simulink model "Boat_sim"  (Simulink 7.8)
settings: Solver=FixedStepDiscrete  StartTime=0.0  StopTime=1000  FixedStep=.01  RelTol=1e-3
InitFcn:
  | clear all
  | missions
  | common
  | physical_constants
  | simulation_constants
  | initial_values
  | l2plus
values from neighbouring files (symbols this model uses):
  InitialPoint = 0    [l2plus.m]
  IPStar = 0    [l2plus.m]
  MaxDwnPthStar = 1    [l2plus.m]
  OC2max = 49999    [simulation_constants.m]
  phi_0 = 0    [simulation_constants.m]
  switchDistance = 4    [l2plus.m]
  T_step = 0.01    [common.m]
  tanIntercept = tan( 45*pi/180 )    [l2plus.m]
  TStar = single(4.5)    [l2plus.m]
  Turn2Track = 0    [l2plus.m]
  wheelbase = 3.27    [physical_constants.m]
undefined symbols (not defined in the file or in its folder): DiscIntNeverNeededParam, Earth, figure8_waypoints, sampling_waypoints, test_waypoints, WGS84
libraries: simulink x21, uSimLib x21, instrumentlib x2, aerolibtransform2 x1, aerolibanimutils x1, simulink_need_slupdate x1
(part 1 of 2)
settings Model: Creator=Administrator  LastModifiedBy=Bryant  ExtModeAutoUpdateStatusClock=off  BufferReuse=off
settings DataIOCC: MaxDataPoints=1  SaveOutput=off  SignalLogging=off
settings OptimizationCC: BlockReduction=off  InlineParams=on  UseIntDivNetSlope=on  InlineInvariantSignals=on  BufferReuse=off  InitFltsAndDblsToZero=on  EfficientFloat2IntCast=on  SimCompilerOptimization=On
settings DebuggingCC: ReadBeforeWriteMsg=DisableAll  SaveWithParameterizedLinksMsg=none  UnderspecifiedInitializationDetection=Simplified  UniqueDataStoreMsg=error  AssertControl=DisableAll
settings HardwareCC: ProdBitPerInt=16  ProdBitPerPointer=16  ProdIntDivRoundTo=Zero  ProdEndianess=LittleEndian  ProdWordSize=16  ProdHWDeviceType=Microchip->dsPIC
settings SFSimCC: SimParseCustomCode=off
settings GRTTargetCC: TargetFcnLib=ansi_tfl_tmw.mat

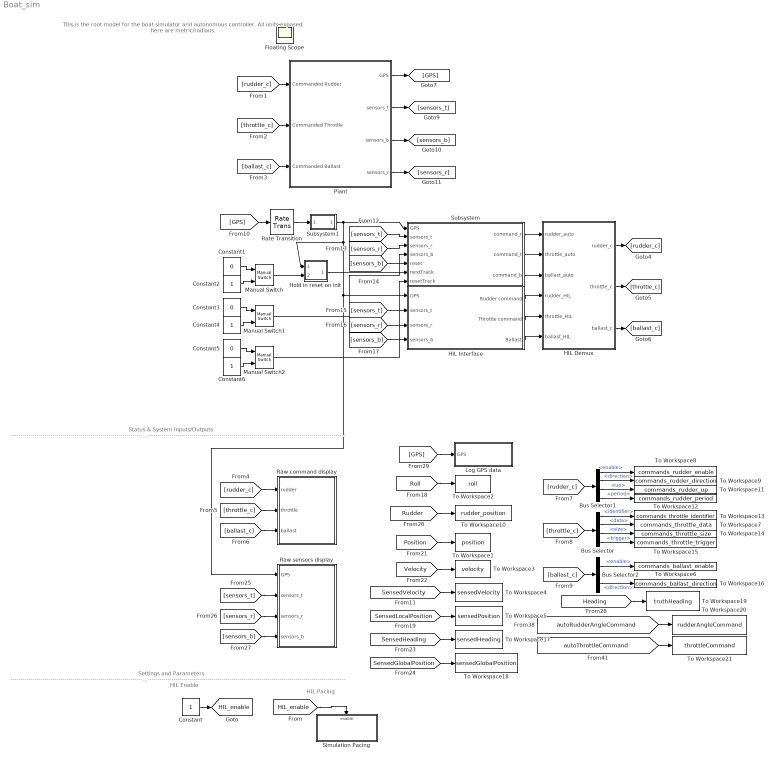
== system Boat_sim ==
  note: This is the root model for the boat simulator and autonomous controller. All
      | units exposed here are metric/radians.
  note: HIL Enable
  note: Settings and Parameters
      | ---------------------------------------------------------------------------------------------------------------------------------------------------------------------------------------------------------------------------------------------------------
  note: HIL Pacing
  note: Status & System Inputs/Outputs
      | ---------------------------------------------------------------------------------------------------------------------------------------------------------------------------------------------------------------------------------------------------------
  Bus Selector : BusSelector  OutputSignals=identifier,data,size,trigger
  Bus Selector1 : BusSelector  OutputSignals=enable,direction,up,period
  Bus Selector2 : BusSelector  OutputSignals=enable,direction
  Constant : Constant  OutDataTypeStr=boolean
  Constant1 : Constant  Value=0  OutDataTypeStr=boolean  SampleTime=Inf
  Constant2 : Constant  OutDataTypeStr=boolean  SampleTime=Inf
  Constant3 : Constant  Value=0  OutDataTypeStr=boolean  SampleTime=Inf
  Constant4 : Constant  OutDataTypeStr=boolean  SampleTime=Inf
  Constant5 : Constant  Value=0  OutDataTypeStr=boolean  SampleTime=Inf
  Constant6 : Constant  OutDataTypeStr=boolean  SampleTime=Inf
  HIL Demux : Subsystem
  HIL Interface : Subsystem
  Hold in reset on init : Subsystem
  Log GPS data : Subsystem
  Manual Switch : simulink/Signal Routing/Manual Switch  sw=1  action=0  varsize=off
  Manual Switch1 : simulink/Signal Routing/Manual Switch  sw=1  action=0  varsize=off
  Manual Switch2 : simulink/Signal Routing/Manual Switch  sw=1  action=0  varsize=off
  Plant : Subsystem
  Rate Transition : RateTransition  OutPortSampleTime=T_step
  Raw command display : Subsystem
  Raw sensors display : Subsystem
  Simulation Pacing : Subsystem  TreatAsAtomicUnit=on
  Subsystem : Subsystem
  Subsystem1 : Subsystem
  To Workspace1 : ToWorkspace  VariableName=position  SampleTime=-1  SaveFormat=Array
  To Workspace10 : ToWorkspace  VariableName=rudder_position  SampleTime=-1  SaveFormat=Array
  To Workspace11 : ToWorkspace  VariableName=commands_rudder_up  SampleTime=-1  SaveFormat=Array
  To Workspace12 : ToWorkspace  VariableName=commands_rudder_period  SampleTime=-1  SaveFormat=Array
  To Workspace13 : ToWorkspace  VariableName=commands_throttle_identifier  SampleTime=-1  SaveFormat=Array
  To Workspace14 : ToWorkspace  VariableName=commands_throttle_size  SampleTime=-1  SaveFormat=Array
  To Workspace15 : ToWorkspace  VariableName=commands_throttle_trigger  SampleTime=-1  SaveFormat=Array
  To Workspace16 : ToWorkspace  VariableName=commands_ballast_direction  SampleTime=-1  SaveFormat=Array
  To Workspace17 : ToWorkspace  VariableName=sensedHeading  SampleTime=-1  SaveFormat=Array
  To Workspace18 : ToWorkspace  VariableName=sensedGlobalPosition  SampleTime=-1  SaveFormat=Array
  To Workspace19 : ToWorkspace  VariableName=truthHeading  SampleTime=-1  SaveFormat=Array
  To Workspace2 : ToWorkspace  VariableName=roll  SampleTime=-1  SaveFormat=Array
  To Workspace20 : ToWorkspace  VariableName=rudderAngleCommand  SampleTime=-1  SaveFormat=Array
  To Workspace21 : ToWorkspace  VariableName=throttleCommand  SampleTime=-1  SaveFormat=Array
  To Workspace3 : ToWorkspace  VariableName=velocity  SampleTime=-1  SaveFormat=Array
  To Workspace4 : ToWorkspace  VariableName=sensedVelocity  SampleTime=-1  SaveFormat=Array
  To Workspace5 : ToWorkspace  VariableName=sensedPosition  SampleTime=-1  SaveFormat=Array
  To Workspace6 : ToWorkspace  VariableName=commands_ballast_enable  SampleTime=-1  SaveFormat=Array
  To Workspace7 : ToWorkspace  VariableName=commands_throttle_data  SampleTime=-1  SaveFormat=Array
  To Workspace8 : ToWorkspace  VariableName=commands_rudder_enable  SampleTime=-1  SaveFormat=Array
  To Workspace9 : ToWorkspace  VariableName=commands_rudder_direction  SampleTime=-1  SaveFormat=Array
  Floating Scope : Scope
      settings: Floating=on
  tag scope: HIL_enable=global
  wires:
  Plant/4(sensors_r) -> [sensors_r]
  Constant/1 -> [HIL_enable]
  Subsystem/1(command_r) -> HIL Demux/1(rudder_auto)
  Subsystem/2(command_t) -> HIL Demux/2(throttle_auto)
  Subsystem/3(command_b) -> HIL Demux/3(ballast_auto)
  [rudder_c] -> Plant/1(Commanded Rudder)
  [throttle_c] -> Plant/2(Commanded Throttle)
  [ballast_c] -> Plant/3(Commanded Ballast)
  Plant/1(GPS) -> [GPS]
  Plant/3(sensors_b) -> [sensors_b]
  Plant/2(sensors_t) -> [sensors_t]
  [sensors_b] -> Subsystem/4(sensors_b)
  [sensors_r] -> Subsystem/3(sensors_r)
  [sensors_t] -> Subsystem/2(sensors_t)
  Constant1/1 -> Manual Switch/1
  Constant2/1 -> Manual Switch/2
  [rudder_c] -> Raw command display/1(rudder)
  [throttle_c] -> Raw command display/2(throttle)
  [ballast_c] -> Raw command display/3(ballast)
  [sensors_t] -> Raw sensors display/2(sensors_t)
  [sensors_r] -> Raw sensors display/3(sensors_r)
  [sensors_b] -> Raw sensors display/4(sensors_b)
  HIL Interface/1(Rudder command) -> HIL Demux/4(rudder_HIL)
  HIL Interface/2(Throttle command) -> HIL Demux/5(throttle_HIL)
  HIL Interface/3(Ballast) -> HIL Demux/6(ballast_HIL)
  HIL Demux/1(rudder_c) -> [rudder_c]
  HIL Demux/3(ballast_c) -> [ballast_c]
  HIL Demux/2(throttle_c) -> [throttle_c]
  [sensors_b] -> HIL Interface/4(sensors_b)
  [sensors_r] -> HIL Interface/3(sensors_r)
  [sensors_t] -> HIL Interface/2(sensors_t)
  [HIL_enable] -> Simulation Pacing/Enable
  [ballast_c] -> Bus Selector2/1
  [Roll] -> To Workspace2/1
  [Rudder] -> To Workspace10/1
  [Position] -> To Workspace1/1
  [throttle_c] -> Bus Selector/1
  Bus Selector/2 -> To Workspace7/1  "<data>"
  [rudder_c] -> Bus Selector1/1
  Bus Selector1/1 -> To Workspace8/1  "<enable>"
  [Velocity] -> To Workspace3/1
  Hold in reset on init/1(Out1) -> Subsystem/5(reset)
  Manual Switch/1 -> Hold in reset on init/2(reset)
  [GPS] -> Rate Transition/1
  Subsystem1/1(GPS+newData) -> Subsystem/1(GPS), Hold in reset on init/1(GPS), HIL Interface/1(GPS), Raw sensors display/1(GPS)
  Constant3/1 -> Manual Switch1/1
  Constant4/1 -> Manual Switch1/2
  Constant5/1 -> Manual Switch2/1
  Constant6/1 -> Manual Switch2/2
  Manual Switch2/1 -> Subsystem/7(resetTrack)
  Manual Switch1/1 -> Subsystem/6(nextTrack)
  [SensedVelocity] -> To Workspace4/1
  [SensedLocalPosition] -> To Workspace5/1
  Bus Selector1/2 -> To Workspace9/1  "<direction>"
  Bus Selector1/3 -> To Workspace11/1  "<up>"
  Bus Selector1/4 -> To Workspace12/1  "<period>"
  Bus Selector/1 -> To Workspace13/1  "<identifier>"
  Bus Selector/3 -> To Workspace14/1  "<size>"
  Bus Selector/4 -> To Workspace15/1  "<trigger>"
  Bus Selector2/1 -> To Workspace6/1  "<enable>"
  Bus Selector2/2 -> To Workspace16/1  "<direction>"
  [SensedHeading] -> To Workspace17/1
  [SensedGlobalPosition] -> To Workspace18/1
  [Heading] -> To Workspace19/1
  [autoRudderAngleCommand] -> To Workspace20/1
  [autoThrottleCommand] -> To Workspace21/1
  [GPS] -> Log GPS data/1(GPS)
  Rate Transition/1 -> Subsystem1/1(GPS)

== system Boat_sim/HIL Demux ==
  rudder_auto : Inport
  throttle_auto : Inport  Port=2
  ballast_auto : Inport  Port=3
  rudder_HIL : Inport  Port=4
  throttle_HIL : Inport  Port=5
  ballast_HIL : Inport  Port=6
  Switch : Switch  Criteria=u2 ~= 0
  Switch1 : Switch  Criteria=u2 ~= 0
  Switch2 : Switch  Criteria=u2 ~= 0
  rudder_c : Outport
  throttle_c : Outport  Port=2
  ballast_c : Outport  Port=3
  wires:
  rudder_HIL/1 -> Switch/1
  [HIL_enable] -> Switch/2, Switch1/2, Switch2/2
  throttle_HIL/1 -> Switch1/1
  ballast_HIL/1 -> Switch2/1
  throttle_auto/1 -> Switch1/3
  rudder_auto/1 -> Switch/3
  ballast_auto/1 -> Switch2/3
  Switch/1 -> rudder_c/1
  Switch1/1 -> throttle_c/1
  Switch2/1 -> ballast_c/1

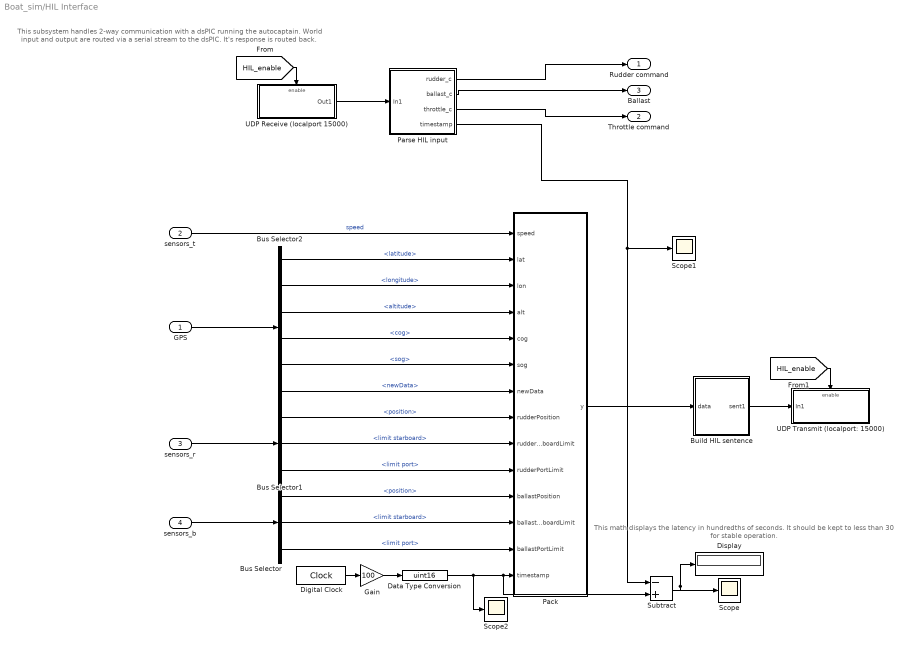
== system Boat_sim/HIL Interface ==
  note: This subsystem handles 2-way communication with a dsPIC running
      | the autocaptain. World input and output are routed via a serial stream
      | to the dsPIC. It's response is routed back.
  note: This math displays the latency in hundredths of seconds.
      | It should be kept to less than 30 for stable operation.
  GPS : Inport
  sensors_t : Inport  Port=2
  sensors_r : Inport  Port=3
  sensors_b : Inport  Port=4
  Build HIL sentence : Subsystem
  Bus Selector : BusSelector  OutputSignals=position,limit starboard,limit port
  Bus Selector1 : BusSelector  OutputSignals=position,limit starboard,limit port
  Bus Selector2 : BusSelector  OutputSignals=latitude,longitude,altitude,cog,sog,newData
  Data Type Conversion : DataTypeConversion  OutDataTypeStr=uint16
  Digital Clock : DigitalClock  SampleTime=.01
  Display : Display
  Gain : Gain  Gain=100
  Pack : MATLAB Function  TreatAsAtomicUnit=on
  Parse HIL input : Subsystem
  Scope : Scope
      settings: YMin=40  YMax=92.5  SaveName=latency  DataFormat=Array
  Scope1 : Scope
      settings: YMin=1470.6  YMax=1625.4  SaveName=latency_in  DataFormat=Array
  Scope2 : Scope
      settings: TimeRange=14  YMin=0  YMax=1400  SaveName=latency_out  DataFormat=Array
  Subtract : Sum  Inputs=-+  OutDataTypeStr=int16
  UDP Receive (localport 15000) : Subsystem  TreatAsAtomicUnit=on
  UDP Transmit (localport: 15000) : Subsystem  TreatAsAtomicUnit=on
  Rudder command : Outport
  Throttle command : Outport  Port=2
  Ballast : Outport  Port=3
  wires:
  UDP Receive (localport 15000)/1(Out1) -> Parse HIL input/1(In1)
  Parse HIL input/2(ballast_c) -> Ballast/1
  Parse HIL input/1(rudder_c) -> Rudder command/1
  sensors_b/1 -> Bus Selector/1
  sensors_r/1 -> Bus Selector1/1
  GPS/1 -> Bus Selector2/1
  Parse HIL input/3(throttle_c) -> Throttle command/1
  Pack/1(y) -> Build HIL sentence/1(data)
  sensors_t/1 -> Pack/1(speed)  "speed"
  Bus Selector2/1 -> Pack/2(lat)  "<latitude>"
  Bus Selector2/2 -> Pack/3(lon)  "<longitude>"
  Bus Selector2/3 -> Pack/4(alt)  "<altitude>"
  Bus Selector2/4 -> Pack/5(cog)  "<cog>"
  Bus Selector2/5 -> Pack/6(sog)  "<sog>"
  [HIL_enable] -> UDP Receive (localport 15000)/Enable
  [HIL_enable] -> UDP Transmit (localport: 15000)/Enable
  Build HIL sentence/1(sent1) -> UDP Transmit (localport: 15000)/1(In1)
  Parse HIL input/4(timestamp) -> Subtract/1, Scope1/1
  Gain/1 -> Data Type Conversion/1
  Digital Clock/1 -> Gain/1
  Data Type Conversion/1 -> Subtract/2, Pack/14(timestamp), Scope2/1
  Subtract/1 -> Scope/1, Display/1
  Bus Selector2/6 -> Pack/7(newData)  "<newData>"
  Bus Selector1/1 -> Pack/8(rudderPosition)  "<position>"
  Bus Selector1/2 -> Pack/9(rudderStarboardLimit)  "<limit starboard>"
  Bus Selector1/3 -> Pack/10(rudderPortLimit)  "<limit port>"
  Bus Selector/1 -> Pack/11(ballastPosition)  "<position>"
  Bus Selector/2 -> Pack/12(ballastStarboardLimit)  "<limit starboard>"
  Bus Selector/3 -> Pack/13(ballastPortLimit)  "<limit port>"

== system Boat_sim/Hold in reset on init ==
  GPS : Inport
  reset : Inport  Port=2
  Bus Selector : BusSelector  OutputSignals=newData
  Compare To Zero : simulink/Logic and Bit Operations/Compare To Zero  relop===  OutDataTypeStr=boolean
  Discrete-Time Integrator : DiscreteIntegrator  SampleTime=-1  LimitOutput=on  UpperSaturationLimit=1  LowerSaturationLimit=0  ICPrevOutput=DiscIntNeverNeededParam  ICPrevScaledInput=DiscIntNeverNeededParam
  Logical Operator : Logic  Operator=OR  AllPortsSameDT=off  OutDataTypeStr=boolean
  Out1 : Outport
  wires:
  Bus Selector/1 -> Discrete-Time Integrator/1  "<newData>"
  Discrete-Time Integrator/1 -> Compare To Zero/1
  Compare To Zero/1 -> Logical Operator/1
  GPS/1 -> Bus Selector/1
  Logical Operator/1 -> Out1/1
  reset/1 -> Logical Operator/2

== system Boat_sim/Log GPS data ==
  GPS : Inport
  Bus Selector3 : BusSelector  OutputSignals=latitude,longitude,altitude,cog,sog
  Mux : Mux  Inputs=3
  To Workspace28 : ToWorkspace  VariableName=globalPosition  SampleTime=-1  SaveFormat=Array
  To Workspace29 : ToWorkspace  VariableName=courseOverGround  SampleTime=-1  SaveFormat=Array
  To Workspace30 : ToWorkspace  VariableName=speedOverGround  SampleTime=-1  SaveFormat=Array
  wires:
  Mux/1 -> To Workspace28/1
  Bus Selector3/1 -> Mux/1  "<latitude>"
  Bus Selector3/2 -> Mux/2  "<longitude>"
  Bus Selector3/3 -> Mux/3  "<altitude>"
  Bus Selector3/4 -> To Workspace29/1  "<cog>"
  Bus Selector3/5 -> To Workspace30/1  "<sog>"
  GPS/1 -> Bus Selector3/1

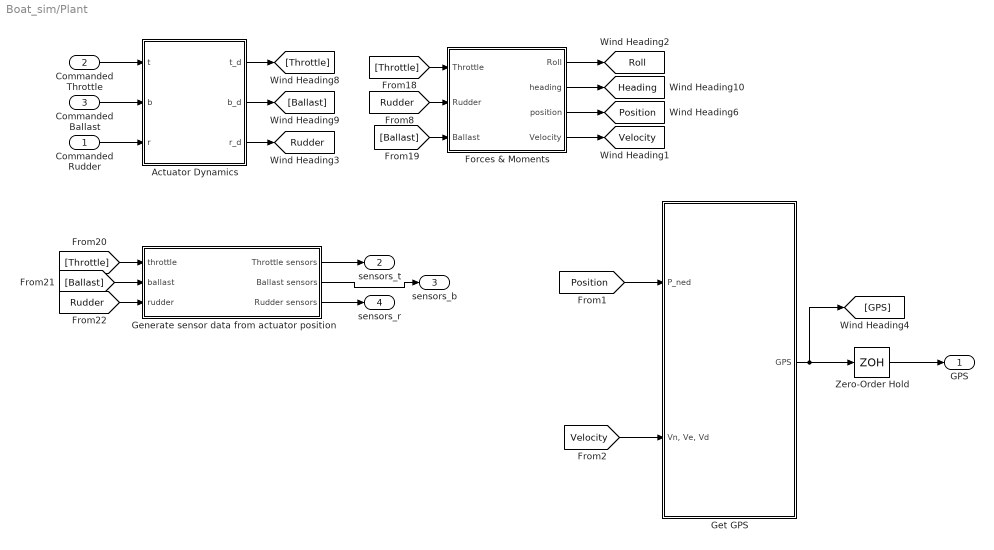
== system Boat_sim/Plant ==
  Commanded Rudder : Inport
  Commanded Throttle : Inport  Port=2
  Commanded Ballast : Inport  Port=3
  Actuator Dynamics : Subsystem
  Forces & Moments : Subsystem
  Generate sensor data from actuator position : Subsystem
  Get GPS : Subsystem
  Zero-Order Hold : ZeroOrderHold  SampleTime=.2
  GPS : Outport
  sensors_t : Outport  Port=2
  sensors_b : Outport  Port=3
  sensors_r : Outport  Port=4
  tag scope: Heading=global, Position=global, Roll=global, Rudder=global, Velocity=global
  wires:
  Commanded Throttle/1 -> Actuator Dynamics/1(t)
  Commanded Rudder/1 -> Actuator Dynamics/3(r)
  Forces & Moments/1(Roll) -> [Roll]
  Commanded Ballast/1 -> Actuator Dynamics/2(b)
  Actuator Dynamics/3(r_d) -> [Rudder]
  [Rudder] -> Forces & Moments/2(Rudder)
  Actuator Dynamics/1(t_d) -> [Throttle]
  [Throttle] -> Forces & Moments/1(Throttle)
  [Ballast] -> Forces & Moments/3(Ballast)
  Actuator Dynamics/2(b_d) -> [Ballast]
  Forces & Moments/2(heading) -> [Heading]
  [Position] -> Get GPS/1(P_ned)
  [Velocity] -> Get GPS/2("Vn, Ve, Vd")
  Get GPS/1(GPS) -> [GPS], Zero-Order Hold/1
  [Rudder] -> Generate sensor data from actuator position/3(rudder)
  [Ballast] -> Generate sensor data from actuator position/2(ballast)
  [Throttle] -> Generate sensor data from actuator position/1(throttle)
  Generate sensor data from actuator position/1(Throttle sensors) -> sensors_t/1
  Generate sensor data from actuator position/2(Ballast sensors) -> sensors_b/1
  Generate sensor data from actuator position/3(Rudder sensors) -> sensors_r/1
  Forces & Moments/4(Velocity) -> [Velocity]
  Forces & Moments/3(position) -> [Position]
  Zero-Order Hold/1 -> GPS/1

== system Boat_sim/Raw command display ==
  rudder : Inport
  throttle : Inport  Port=2
  ballast : Inport  Port=3
  Bus Selector3 : BusSelector  OutputSignals=enable,direction,up,period
  Bus Selector4 : BusSelector  OutputSignals=identifier,data,size,trigger
  Bus Selector5 : BusSelector  OutputSignals=enable,direction
  Display{,1..9} (10 alike) : Display
      Display4 settings: Format=hex (Stored Integer)
      Display5 settings: Format=hex (Stored Integer)
  wires:
  Bus Selector3/4 -> Display3/1  "<period>"
  Bus Selector3/1 -> Display/1  "<enable>"
  Bus Selector3/2 -> Display1/1  "<direction>"
  Bus Selector3/3 -> Display2/1  "<up>"
  Bus Selector4/4 -> Display7/1  "<trigger>"
  Bus Selector4/1 -> Display4/1  "<identifier>"
  Bus Selector4/2 -> Display5/1  "<data>"
  Bus Selector4/3 -> Display6/1  "<size>"
  Bus Selector5/2 -> Display8/1  "<direction>"
  Bus Selector5/1 -> Display9/1  "<enable>"
  rudder/1 -> Bus Selector3/1
  throttle/1 -> Bus Selector4/1
  ballast/1 -> Bus Selector5/1

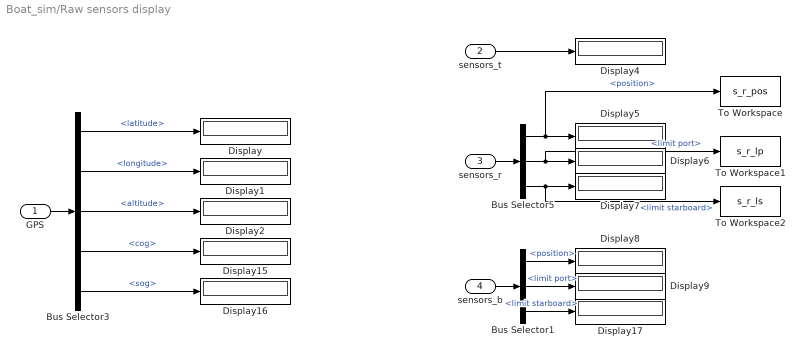
== system Boat_sim/Raw sensors display ==
  GPS : Inport
  sensors_t : Inport  Port=2
  sensors_r : Inport  Port=3
  sensors_b : Inport  Port=4
  Bus Selector1 : BusSelector  OutputSignals=position,limit port,limit starboard
  Bus Selector3 : BusSelector  OutputSignals=latitude,longitude,altitude,cog,sog
  Bus Selector5 : BusSelector  OutputSignals=position,limit port,limit starboard
  Display{,1..2,4..9,15..17} (12 alike) : Display
  To Workspace : ToWorkspace  VariableName=s_r_pos  SampleTime=-1  SaveFormat=Array
  To Workspace1 : ToWorkspace  VariableName=s_r_lp  SampleTime=-1  SaveFormat=Array
  To Workspace2 : ToWorkspace  VariableName=s_r_ls  SampleTime=-1  SaveFormat=Array
  wires:
  Bus Selector3/1 -> Display/1  "<latitude>"
  Bus Selector3/2 -> Display1/1  "<longitude>"
  Bus Selector3/3 -> Display2/1  "<altitude>"
  GPS/1 -> Bus Selector3/1
  sensors_t/1 -> Display4/1
  sensors_r/1 -> Bus Selector5/1
  Bus Selector3/4 -> Display15/1  "<cog>"
  Bus Selector3/5 -> Display16/1  "<sog>"
  sensors_b/1 -> Bus Selector1/1
  Bus Selector5/1 -> Display5/1, To Workspace/1  "<position>"
  Bus Selector5/2 -> Display6/1, To Workspace1/1  "<limit port>"
  Bus Selector5/3 -> Display7/1, To Workspace2/1  "<limit starboard>"
  Bus Selector1/1 -> Display8/1  "<position>"
  Bus Selector1/2 -> Display9/1  "<limit port>"
  Bus Selector1/3 -> Display17/1  "<limit starboard>"

== system Boat_sim/Simulation Pacing ==
  note: This block attempts to lock the simulation down to real-time. This does, however, require that the sim run faster than real time originally,
      | then the Set Pace block sleeps the MATLAB  process to fill up the time til it paces realtime. The number in the display block shouldn't be
      | far from 0 and will probably bounce around both above and below. If it stays substantially below zero (<-.01), then there's a problem as
      | the sim isn't keeping time.
  Enable : EnablePort
  Display1 : Display
      settings: Decimation=20
  Scope : Scope
      settings: SaveName=paceError  DataFormat=Array
  Simulation Pace : aerolibanimutils/Simulation Pace  SimulationPace=1  SleepMode=MATLAB Thread  OutputPaceError=on  SampleTime=T_step
      settings: AttributesFormatString=%<SimulationPace> sec/sec
  wires:
  Simulation Pace/1 -> Display1/1, Scope/1

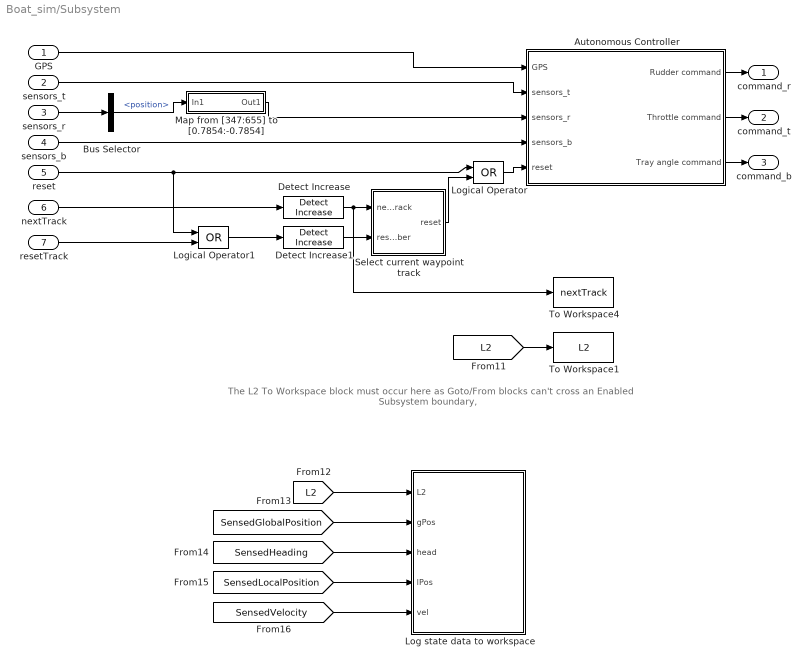
== system Boat_sim/Subsystem ==
  note: The L2 To Workspace block must occur here
      | as Goto/From blocks can't cross an Enabled
      | Subsystem boundary,
  GPS : Inport
  sensors_t : Inport  Port=2
  sensors_r : Inport  Port=3
  sensors_b : Inport  Port=4
  reset : Inport  Port=5
  nextTrack : Inport  Port=6
  resetTrack : Inport  Port=7
  Autonomous Controller : Subsystem  Priority=1
  Bus Selector : BusSelector  OutputSignals=position
  Detect Increase : simulink/Logic and Bit Operations/Detect Increase  vinit=0.0  InputProcessing=Inherited  OutDataTypeStr=boolean
  Detect Increase1 : simulink/Logic and Bit Operations/Detect Increase  vinit=0.0  InputProcessing=Inherited  OutDataTypeStr=boolean
  Log state data to workspace : Subsystem
  Logical Operator : Logic  Operator=OR  AllPortsSameDT=off  OutDataTypeStr=boolean
  Logical Operator1 : Logic  Operator=OR  AllPortsSameDT=off  OutDataTypeStr=boolean
  Map from [347:655] to [0.7854:-0.7854] : Subsystem
  Select current waypoint track : MATLAB Function  TreatAsAtomicUnit=on
  To Workspace1 : ToWorkspace  VariableName=L2  SampleTime=-1  SaveFormat=Array
  To Workspace4 : ToWorkspace  VariableName=nextTrack  SampleTime=-1  SaveFormat=Array
  command_r : Outport
  command_t : Outport  Port=2
  command_b : Outport  Port=3
  wires:
  GPS/1 -> Autonomous Controller/1(GPS)
  Autonomous Controller/1(Rudder command) -> command_r/1
  sensors_t/1 -> Autonomous Controller/2(sensors_t)
  sensors_r/1 -> Bus Selector/1
  Autonomous Controller/2(Throttle command) -> command_t/1
  sensors_b/1 -> Autonomous Controller/4(sensors_b)
  Autonomous Controller/3(Tray angle command) -> command_b/1
  nextTrack/1 -> Detect Increase/1
  Logical Operator/1 -> Autonomous Controller/5(reset)
  Select current waypoint track/1(reset) -> Logical Operator/2
  reset/1 -> Logical Operator/1, Logical Operator1/1
  Detect Increase/1 -> Select current waypoint track/1(nextTrack), To Workspace4/1
  Detect Increase1/1 -> Select current waypoint track/2(resetTrackNumber)
  [L2] -> To Workspace1/1
  Logical Operator1/1 -> Detect Increase1/1
  resetTrack/1 -> Logical Operator1/2
  [SensedVelocity] -> Log state data to workspace/5(vel)
  [L2] -> Log state data to workspace/1(L2)
  [SensedGlobalPosition] -> Log state data to workspace/2(gPos)
  [SensedHeading] -> Log state data to workspace/3(head)
  [SensedLocalPosition] -> Log state data to workspace/4(lPos)
  Map from [347:655] to [0.7854:-0.7854]/1(Out1) -> Autonomous Controller/3(sensors_r)
  Bus Selector/1 -> Map from [347:655] to [0.7854:-0.7854]/1(In1)  "<position>"

== system Boat_sim/Subsystem1 ==
  GPS : Inport
  Bus Assignment : BusAssignment  AssignedSignals=newData
  Data Type Conversion : DataTypeConversion  OutDataTypeStr=boolean
  Pulse Generator : DiscretePulseGenerator  Period=20  PhaseDelay=100  SampleTime=T_step
  GPS+newData : Outport
  wires:
  Pulse Generator/1 -> Data Type Conversion/1
  Data Type Conversion/1 -> Bus Assignment/2
  GPS/1 -> Bus Assignment/1
  Bus Assignment/1 -> GPS+newData/1

== system Boat_sim/HIL Interface/Build HIL sentence ==
  data : Inport
  Bitwise Operator1 : simulink/Logic and Bit Operations/Bitwise Operator  logicop=XOR  UseBitMask=off  BitMask=bin2dec('11011001')  BitMaskRealWorld=Stored Integer
  Constant5 : Constant  Value=37  OutDataTypeStr=uint8
  Constant6 : Constant  Value=38  OutDataTypeStr=uint8
  Constant7 : Constant  Value=94  OutDataTypeStr=uint8
  Constant8 : Constant  Value=38  OutDataTypeStr=uint8
  Constant9 : Constant  OutDataTypeStr=uint8
  Mux3 : Mux  Inputs=3
  Pack : MATLAB Function  TreatAsAtomicUnit=on
  Probe : Probe  ProbeSampleTime=off  ProbeComplexSignal=off  ProbeWidthDataType=uint8
  sent1 : Outport
  wires:
  data/1 -> Probe/1, Mux3/3
  Constant5/1 -> Pack/1(a)
  Constant6/1 -> Pack/2(b)
  Pack/1(y) -> sent1/1
  Mux3/1 -> Bitwise Operator1/1, Pack/3(c)
  Probe/1 -> Mux3/2
  Constant7/1 -> Pack/4(d)
  Constant8/1 -> Pack/5(e)
  Bitwise Operator1/1 -> Pack/6(f)
  Constant9/1 -> Mux3/1

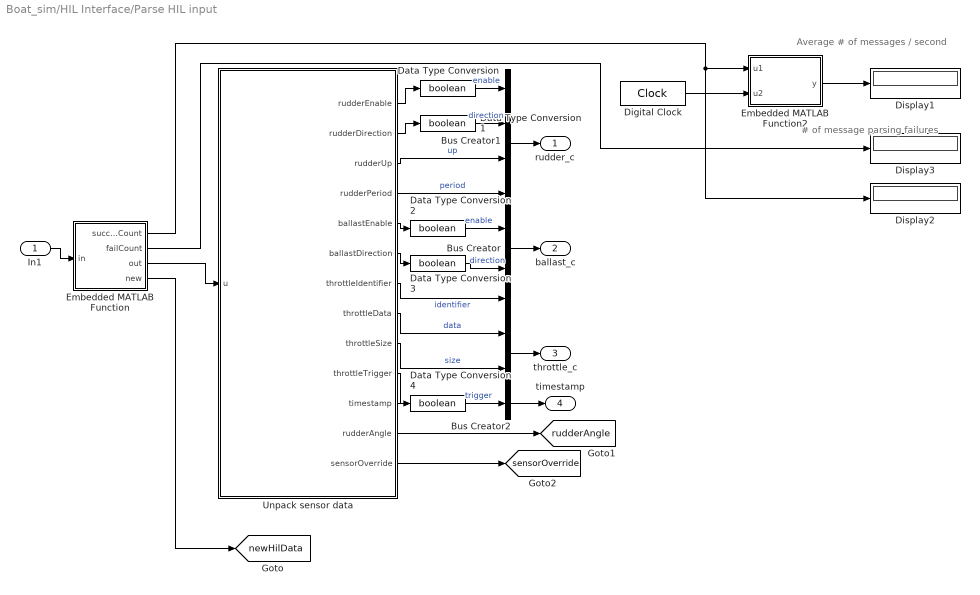
== system Boat_sim/HIL Interface/Parse HIL input ==
  note: # of message parsing failures
  note: Average # of messages / second
  In1 : Inport
  Bus Creator : BusCreator  Inputs=2
  Bus Creator1 : BusCreator
  Bus Creator2 : BusCreator
  Data Type Conversion{,1..4} (5 alike) : DataTypeConversion  OutDataTypeStr=boolean
  Digital Clock : DigitalClock  SampleTime=T_step
  Display1 : Display
  Display2 : Display
  Display3 : Display
  Embedded MATLAB Function : MATLAB Function  TreatAsAtomicUnit=on
  Embedded MATLAB Function2 : MATLAB Function  TreatAsAtomicUnit=on
  Unpack sensor data : MATLAB Function  TreatAsAtomicUnit=on
  rudder_c : Outport
  ballast_c : Outport  Port=2
  throttle_c : Outport  Port=3
  timestamp : Outport  Port=4
  tag scope: newHilData=global, rudderAngle=global, sensorOverride=global
  wires:
  Embedded MATLAB Function/3(out) -> Unpack sensor data/1(u)
  Bus Creator1/1 -> rudder_c/1
  In1/1 -> Embedded MATLAB Function/1(in)
  Bus Creator/1 -> ballast_c/1
  Bus Creator2/1 -> throttle_c/1
  Unpack sensor data/1(rudderEnable) -> Data Type Conversion/1
  Unpack sensor data/2(rudderDirection) -> Data Type Conversion1/1
  Unpack sensor data/3(rudderUp) -> Bus Creator1/3  "up"
  Unpack sensor data/4(rudderPeriod) -> Bus Creator1/4  "period"
  Unpack sensor data/5(ballastEnable) -> Data Type Conversion2/1
  Unpack sensor data/6(ballastDirection) -> Data Type Conversion3/1
  Unpack sensor data/7(throttleIdentifier) -> Bus Creator2/1  "identifier"
  Unpack sensor data/8(throttleData) -> Bus Creator2/2  "data"
  Unpack sensor data/9(throttleSize) -> Bus Creator2/3  "size"
  Unpack sensor data/10(throttleTrigger) -> Data Type Conversion4/1
  Unpack sensor data/11(timestamp) -> timestamp/1
  Embedded MATLAB Function/1(successCount) -> Embedded MATLAB Function2/1(u1), Display2/1
  Digital Clock/1 -> Embedded MATLAB Function2/2(u2)
  Embedded MATLAB Function2/1(y) -> Display1/1
  Data Type Conversion/1 -> Bus Creator1/1  "enable"
  Data Type Conversion1/1 -> Bus Creator1/2  "direction"
  Data Type Conversion2/1 -> Bus Creator/1  "enable"
  Data Type Conversion3/1 -> Bus Creator/2  "direction"
  Data Type Conversion4/1 -> Bus Creator2/4  "trigger"
  Embedded MATLAB Function/2(failCount) -> Display3/1
  Unpack sensor data/12(rudderAngle) -> [rudderAngle]
  Embedded MATLAB Function/4(new) -> [newHilData]
  Unpack sensor data/13(sensorOverride) -> [sensorOverride]

== system Boat_sim/HIL Interface/UDP Receive (localport 15000) ==
  Enable : EnablePort
  IC : InitialCondition  Value=zeros(34, 1, 'uint8')
  Terminator : Terminator
  UDP Receive : instrumentlib/UDP Receive  Host=127.0.0.1  Port=15000  LocalPort=16000  DataSize=34  EnableBlockingMode=off  Timeout=10  SampleTime=0.01  DataType=uint8  ByteOrder=BigEndian
  Out1 : Outport  SourceOfInitialOutputValue=Input signal
  wires:
  UDP Receive/1 -> IC/1
  UDP Receive/2 -> Terminator/1
  IC/1 -> Out1/1

== system Boat_sim/HIL Interface/UDP Transmit (localport: 15000) ==
  note: This subsystem transmits the necessary data to the dsPIC.
  In1 : Inport
  Enable : EnablePort
  UDP Send : instrumentlib/UDP Send  Host=127.0.0.1  Port=15000  LocalPort=16000  EnableBlockingMode=on  ByteOrder=BigEndian
  wires:
  In1/1 -> UDP Send/1

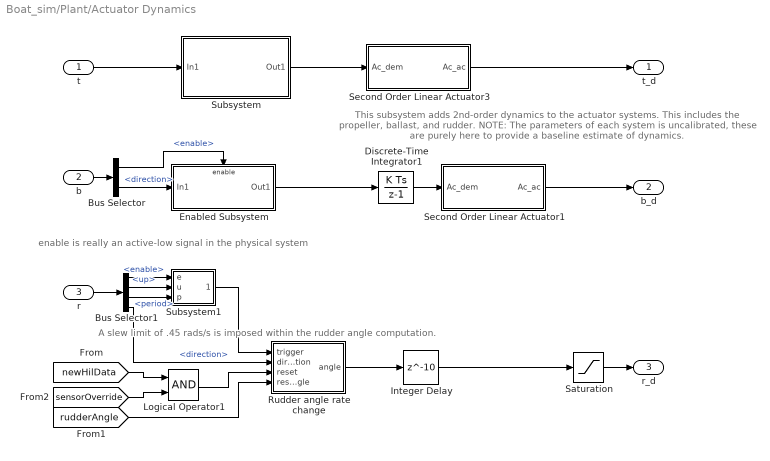
== system Boat_sim/Plant/Actuator Dynamics ==
  note: This subsystem adds 2nd-order dynamics to the actuator systems.
      | This includes the propeller, ballast, and rudder.
      |
      | NOTE: The parameters of each system is uncalibrated, these are
      | purely here to provide a baseline estimate of dynamics.
  note: enable is really an active-low signal
      | in the physical system
  note: A slew limit of .45 rads/s is imposed within the
      | rudder angle computation.
  t : Inport
  b : Inport  Port=2
  r : Inport  Port=3
  Bus Selector : BusSelector  OutputSignals=enable,direction
  Bus Selector1 : BusSelector  OutputSignals=enable,up,period,direction
  Discrete-Time Integrator1 : DiscreteIntegrator  SampleTime=-1  UpperSaturationLimit=1  LowerSaturationLimit=-1  ICPrevOutput=DiscIntNeverNeededParam  ICPrevScaledInput=DiscIntNeverNeededParam
  Enabled Subsystem : Subsystem  TreatAsAtomicUnit=on
  Integer Delay : Delay  DelayLength=10  InputProcessing=Inherited  SampleTime=.01
  Logical Operator1 : Logic  AllPortsSameDT=off  OutDataTypeStr=boolean
  Rudder angle rate change : MATLAB Function  TreatAsAtomicUnit=on
  Saturation : Saturate  UpperLimit=.7854  LowerLimit=-.7854
  Second Order Linear Actuator1 : Subsystem  AncestorBlock=aerolibactuator/Second Order Linear Actuator  mask(Second Order Linear Actuator){wn_fin=15, z_fin=0.8, fin_act_0=0}
      mask prompts: wn_fin "Natural frequency:"; z_fin "Damping ratio:"; fin_act_0 "Initial position:"
      mask help: Implement a second-order actuator model
      mask init:
      | aeroicon('aeroblk');
      mask Help: eval('asbhelp');
      mask Display:
      | port_label('input',1,'A_{demand}','texmode','on');
      | port_label('output',1,'A_{actual}','texmode','on');
  Second Order Linear Actuator3 : Subsystem  AncestorBlock=aerolibactuator/Second Order Linear Actuator  mask(Second Order Linear Actuator){wn_fin=15, z_fin=0.8, fin_act_0=0}
      mask prompts: wn_fin "Natural frequency:"; z_fin "Damping ratio:"; fin_act_0 "Initial position:"
      mask help: Implement a second-order actuator model
      mask init:
      | aeroicon('aeroblk');
      mask Help: eval('asbhelp');
      mask Display:
      | port_label('input',1,'A_{demand}','texmode','on');
      | port_label('output',1,'A_{actual}','texmode','on');
  Subsystem : Subsystem
  Subsystem1 : Subsystem
  t_d : Outport
  b_d : Outport  Port=2
  r_d : Outport  Port=3
  wires:
  r/1 -> Bus Selector1/1
  Second Order Linear Actuator1/1(Ac_ac) -> b_d/1
  Rudder angle rate change/1(angle) -> Integer Delay/1
  Subsystem/1(Out1) -> Second Order Linear Actuator3/1(Ac_dem)
  b/1 -> Bus Selector/1
  Enabled Subsystem/1(Out1) -> Discrete-Time Integrator1/1
  Discrete-Time Integrator1/1 -> Second Order Linear Actuator1/1(Ac_dem)
  Bus Selector/1 -> Enabled Subsystem/Enable  "<enable>"
  Bus Selector/2 -> Enabled Subsystem/1(In1)  "<direction>"
  Bus Selector1/4 -> Rudder angle rate change/2(direction)  "<direction>"
  Bus Selector1/1 -> Subsystem1/1(e)  "<enable>"
  t/1 -> Subsystem/1(In1)
  Bus Selector1/2 -> Subsystem1/2(u)  "<up>"
  Bus Selector1/3 -> Subsystem1/3(p)  "<period>"
  Subsystem1/1(Out1) -> Rudder angle rate change/1(trigger)
  [rudderAngle] -> Rudder angle rate change/4(resetToAngle)
  [newHilData] -> Logical Operator1/1
  [sensorOverride] -> Logical Operator1/2
  Logical Operator1/1 -> Rudder angle rate change/3(reset)
  Second Order Linear Actuator3/1(Ac_ac) -> t_d/1
  Saturation/1 -> r_d/1
  Integer Delay/1 -> Saturation/1

== system Boat_sim/Plant/Forces & Moments ==
  note: This subsystem computes the forward force, heading and roll of the boat that
      | is to be expected based on the current state. The model for these calculations
      | is based off of the calculations performed in the original WG1 boat model.
      |
      | The eventual goal of this subsystem to provide all 6 forces and moments for the
      | boat, instead of only one + final orientation parameters.
  Throttle : Inport
  Rudder : Inport  Port=2
  Ballast : Inport  Port=3
  Convert actuator data to heading and speed : Subsystem
  Initial heading1 : Constant  Value=0
  Subsystem : Subsystem
  Terminator : Terminator
  Roll : Outport
  heading : Outport  Port=2
  position : Outport  Port=3
  Velocity : Outport  Port=4
  wires:
  Throttle/1 -> Convert actuator data to heading and speed/1(Throttle)
  Rudder/1 -> Convert actuator data to heading and speed/2(RudderAngle)
  Ballast/1 -> Terminator/1
  Initial heading1/1 -> Roll/1
  Convert actuator data to heading and speed/2(Heading) -> heading/1, Subsystem/2(Heading)
  Subsystem/1(Position) -> position/1
  Convert actuator data to heading and speed/1(Speed) -> Subsystem/1(Speed)
  Subsystem/2(Velocity) -> Velocity/1

== system Boat_sim/Plant/Generate sensor data from actuator position ==
  note: Rudder sensor data is generated here. Given the ADC configuration onboard the dsPIC
      | as well as the range of voltage values for the rudder pot. the output range should be
      | <=313 for starboard, >=620 for port, and 475<=center<=505. It's mapped from the -+.7854
      | (45deg) range that is used in calculations. The rudder follow the standard right-hand-rule
      | convention and as such +1 corresponds to port and -1 corresponds to starboard.
  note: Limits are set to within 2.5% of the real physical limits. This should
      | provide enough buffer for the real system to handle it. These might want to be changed
      | to actually be closer to the real limit. The potentiometer data gives the controller a good
      | sense of where the actuators are so the limits are just emergency triggers.
  throttle : Inport
  ballast : Inport  Port=2
  rudder : Inport  Port=3
  Bus Creator : BusCreator  Inputs=3
  Bus Creator1 : BusCreator  Inputs=3
  Compare To Constant : simulink/Logic and Bit Operations/Compare To Constant  relop=>=  const=.975  OutDataTypeStr=boolean
  Compare To Constant1 : simulink/Logic and Bit Operations/Compare To Constant  relop=<=  const=-.975  OutDataTypeStr=boolean
  Compare To Constant2 : simulink/Logic and Bit Operations/Compare To Constant  relop=<  const=363  OutDataTypeStr=boolean
  Compare To Constant3 : simulink/Logic and Bit Operations/Compare To Constant  relop=>  const=638  OutDataTypeStr=boolean
  Map from +-.7854 to [347:655] : Subsystem
  Map from -1..1 to -1023..1023 : Subsystem
  Map from -1..1 to 620..313 : Subsystem
  Throttle sensors : Outport
  Ballast sensors : Outport  Port=2
  Rudder sensors : Outport  Port=3
  wires:
  throttle/1 -> Map from -1..1 to -1023..1023/1(In1)
  Bus Creator/1 -> Ballast sensors/1
  Compare To Constant1/1 -> Bus Creator/3  "limit starboard"
  Compare To Constant/1 -> Bus Creator/2  "limit port"
  ballast/1 -> Map from -1..1 to 620..313/1(In1), Compare To Constant/1, Compare To Constant1/1
  Bus Creator1/1 -> Rudder sensors/1
  Compare To Constant3/1 -> Bus Creator1/3  "limit starboard"
  Compare To Constant2/1 -> Bus Creator1/2  "limit port"
  rudder/1 -> Map from +-.7854 to [347:655]/1(In1)
  Map from +-.7854 to [347:655]/1(Out1) -> Bus Creator1/1, Compare To Constant2/1, Compare To Constant3/1  "position"
  Map from -1..1 to 620..313/1(Out1) -> Bus Creator/1  "position"
  Map from -1..1 to -1023..1023/1(Out1) -> Throttle sensors/1

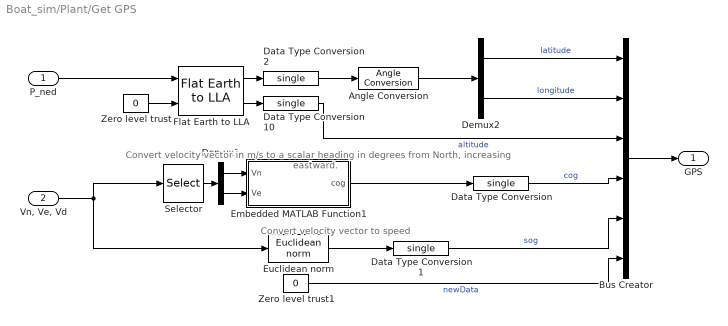
== system Boat_sim/Plant/Get GPS ==
  note: Convert velocity vector to speed
  note: Convert velocity vector in m/s to a scalar heading in degrees from North, increasing eastward.
  P_ned : Inport
  "Vn, Ve, Vd" : Inport  Port=2
  Angle Conversion : uSimLib/Conversions/Angle Conversion  iu=deg  ou=rad
  Bus Creator : BusCreator  Inputs=6  NonVirtualBus=on
  Data Type Conversion{,1..2,10} (4 alike) : DataTypeConversion  OutDataTypeStr=single
  Demux1 : Demux  Outputs=2
  Demux2 : Demux  Outputs=2
  Embedded MATLAB Function1 : MATLAB Function  TreatAsAtomicUnit=on
  Euclidean norm : uSimLib/Math/Euclidean norm  SystemSampleTime=-1
  Flat Earth to LLA : aerolibtransform2/Flat Earth to LLA  units=Metric (MKS)  ptype=Earth (WGS84)  F=1/298.257223563  R=6378137  LL0=initial_LL  psi=0
  Selector : Selector  InputPortWidth=3  IndexOptions=Index vector (dialog)  Indices=[2 1]  OutputSizes=1
  Zero level trust : Constant  Value=0
  Zero level trust1 : Constant  Value=0  OutDataTypeStr=boolean
  GPS : Outport
  wires:
  Zero level trust/1 -> Flat Earth to LLA/2
  P_ned/1 -> Flat Earth to LLA/1
  Flat Earth to LLA/1 -> Data Type Conversion2/1
  Flat Earth to LLA/2 -> Data Type Conversion10/1
  Demux2/1 -> Bus Creator/1  "latitude"
  Demux2/2 -> Bus Creator/2  "longitude"
  Euclidean norm/1 -> Data Type Conversion1/1
  "Vn, Ve, Vd"/1 -> Selector/1, Euclidean norm/1
  Embedded MATLAB Function1/1(cog) -> Data Type Conversion/1
  Bus Creator/1 -> GPS/1
  Data Type Conversion/1 -> Bus Creator/4  "cog"
  Data Type Conversion1/1 -> Bus Creator/5  "sog"
  Data Type Conversion10/1 -> Bus Creator/3  "altitude"
  Selector/1 -> Demux1/1
  Demux1/1 -> Embedded MATLAB Function1/1(Vn)
  Demux1/2 -> Embedded MATLAB Function1/2(Ve)
  Zero level trust1/1 -> Bus Creator/6  "newData"
  Data Type Conversion2/1 -> Angle Conversion/1
  Angle Conversion/1 -> Demux2/1

== system Boat_sim/Subsystem/Autonomous Controller ==
  note: This subsystem currently provides autonomous control of the boat. It utilizes simple PID control
      | on the throttle and rudder based on desired location and bearing. Calculations are performed
      | to compute a straight-line path between current location and the programmed waypoint. The
      | boat then sets out to achieve this course.
  GPS : Inport
  sensors_t : Inport  Port=2
  sensors_r : Inport  Port=3
  sensors_b : Inport  Port=4
  reset : Inport  Port=5
  Ballast Command : Subsystem
  Bus Selector : BusSelector  OutputSignals=sog
  Discrete step : uSimLib/Sources/Discrete step  start_value=1  end_value=0  transition_time=1
  Initialize MissionList : Subsystem  TreatAsAtomicUnit=on
  Rudder Command : Subsystem
  State Keeper & Estimator : Subsystem
  Terminator2 : Terminator
  Throttle Command : Subsystem
  Rudder command : Outport
  Throttle command : Outport  Port=2
  Tray angle command : Outport  Port=3
  wires:
  Discrete step/1 -> Initialize MissionList/Trigger
  reset/1 -> Rudder Command/3(Reset), Throttle Command/2(reset), State Keeper & Estimator/3(reset)
  State Keeper & Estimator/5(pos) -> Rudder Command/4(Local pos)
  State Keeper & Estimator/1(sensors_t) -> Throttle Command/1(sensors)
  State Keeper & Estimator/2(sensors_r) -> Rudder Command/2(Sensors)
  State Keeper & Estimator/4(velocity) -> Rudder Command/1(Velocity)
  GPS/1 -> State Keeper & Estimator/4(gps), Bus Selector/1
  Throttle Command/1(command) -> Throttle command/1
  Rudder Command/1(Command) -> Rudder command/1
  Ballast Command/1(c_ballast) -> Tray angle command/1
  sensors_b/1 -> State Keeper & Estimator/5(ballast)
  sensors_r/1 -> State Keeper & Estimator/2(rudder)
  sensors_t/1 -> State Keeper & Estimator/1(throttle)
  State Keeper & Estimator/3(sensors_b) -> Terminator2/1
  Bus Selector/1 -> Rudder Command/5(Speed)  "<sog>"

== system Boat_sim/Subsystem/Log state data to workspace ==
  L2 : Inport
  gPos : Inport  Port=2
  head : Inport  Port=3
  lPos : Inport  Port=4
  vel : Inport  Port=5
  Build HIL sentence : Subsystem
  Pack : MATLAB Function  TreatAsAtomicUnit=on
  To Workspace2 : ToWorkspace  VariableName=state  SampleTime=-1  SaveFormat=Array
  wires:
  Pack/1(y) -> Build HIL sentence/1(data)
  Build HIL sentence/1(sent) -> To Workspace2/1
  L2/1 -> Pack/1(L2)
  gPos/1 -> Pack/2(gPos)
  head/1 -> Pack/3(head)
  lPos/1 -> Pack/4(lPos)
  vel/1 -> Pack/5(vel)

== system Boat_sim/Subsystem/Map from [347:655] to [0.7854:-0.7854] ==
  In1 : Inport
  Bias1 : Bias  Bias=-501
  Data Type Conversion : DataTypeConversion  OutDataTypeStr=single
  Gain : Gain  Gain=-1/196
  Out1 : Outport
  wires:
  In1/1 -> Data Type Conversion/1
  Gain/1 -> Out1/1
  Bias1/1 -> Gain/1
  Data Type Conversion/1 -> Bias1/1

== system Boat_sim/Plant/Actuator Dynamics/Enabled Subsystem ==
  note: Map from 0,1 to -.02,.02
  In1 : Inport
  Enable : EnablePort
  Bias : Bias  Bias=-1
  Data Type Conversion3 : DataTypeConversion  OutDataTypeStr=single
  Gain : Gain  Gain=2  OutDataTypeStr=double
  Gain1 : Gain  Gain=.05
  IC : InitialCondition  Value=0
  Out1 : Outport  SourceOfInitialOutputValue=Input signal
  wires:
  In1/1 -> Data Type Conversion3/1
  Gain/1 -> Bias/1
  Bias/1 -> Gain1/1
  Gain1/1 -> IC/1
  Data Type Conversion3/1 -> Gain/1
  IC/1 -> Out1/1

== system Boat_sim/Plant/Actuator Dynamics/Second Order Linear Actuator1 ==
  Ac_dem : Inport
  2*zeta * wn : Gain  Gain=2.0 * z_fin* wn_fin  SaturateOnIntegerOverflow=on  OutDataTypeStr=Inherit: Same as input  ParamDataTypeStr=Inherit: Same as input
  Discrete-Time Integrator1 : DiscreteIntegrator  SampleTime=-1  UpperSaturationLimit=1  LowerSaturationLimit=-1  ICPrevOutput=DiscIntNeverNeededParam  ICPrevScaledInput=DiscIntNeverNeededParam
  Discrete-Time Integrator2 : DiscreteIntegrator  SampleTime=-1  UpperSaturationLimit=1  LowerSaturationLimit=-1  ICPrevOutput=DiscIntNeverNeededParam  ICPrevScaledInput=DiscIntNeverNeededParam
  Sum2 : Sum  Inputs=|+-  SaturateOnIntegerOverflow=on  InputSameDT=on  OutDataTypeStr=Inherit: Same as first input
  Sum3 : Sum  Inputs=|+-  SaturateOnIntegerOverflow=on  InputSameDT=on  OutDataTypeStr=Inherit: Same as first input
  wn^2 : Gain  Gain=wn_fin* wn_fin  SaturateOnIntegerOverflow=on  OutDataTypeStr=Inherit: Same as input  ParamDataTypeStr=Inherit: Same as input
  Ac_ac : Outport  InitialOutput=0
  wires:
  Discrete-Time Integrator1/1 -> Ac_ac/1, Sum3/2
  wn^2/1 -> Sum2/1
  Sum2/1 -> Discrete-Time Integrator2/1
  Discrete-Time Integrator2/1 -> 2*zeta * wn/1, Discrete-Time Integrator1/1
  2*zeta * wn/1 -> Sum2/2
  Ac_dem/1 -> Sum3/1
  Sum3/1 -> wn^2/1

== system Boat_sim/Plant/Actuator Dynamics/Second Order Linear Actuator3 ==
  Ac_dem : Inport
  2*zeta * wn : Gain  Gain=2.0 * z_fin* wn_fin  SaturateOnIntegerOverflow=on  OutDataTypeStr=Inherit: Same as input  ParamDataTypeStr=Inherit: Same as input
  Discrete-Time Integrator1 : DiscreteIntegrator  SampleTime=-1  UpperSaturationLimit=1  LowerSaturationLimit=-1  ICPrevOutput=DiscIntNeverNeededParam  ICPrevScaledInput=DiscIntNeverNeededParam
  Discrete-Time Integrator2 : DiscreteIntegrator  SampleTime=-1  UpperSaturationLimit=1  LowerSaturationLimit=-1  ICPrevOutput=DiscIntNeverNeededParam  ICPrevScaledInput=DiscIntNeverNeededParam
  Sum2 : Sum  Inputs=|+-  SaturateOnIntegerOverflow=on  InputSameDT=on  OutDataTypeStr=Inherit: Same as first input
  Sum3 : Sum  Inputs=|+-  SaturateOnIntegerOverflow=on  InputSameDT=on  OutDataTypeStr=Inherit: Same as first input
  wn^2 : Gain  Gain=wn_fin* wn_fin  SaturateOnIntegerOverflow=on  OutDataTypeStr=Inherit: Same as input  ParamDataTypeStr=Inherit: Same as input
  Ac_ac : Outport  InitialOutput=0
  wires:
  Discrete-Time Integrator1/1 -> Ac_ac/1, Sum3/2
  wn^2/1 -> Sum2/1
  Sum2/1 -> Discrete-Time Integrator2/1
  Discrete-Time Integrator2/1 -> 2*zeta * wn/1, Discrete-Time Integrator1/1
  2*zeta * wn/1 -> Sum2/2
  Ac_dem/1 -> Sum3/1
  Sum3/1 -> wn^2/1

== system Boat_sim/Plant/Actuator Dynamics/Subsystem ==
  note: This block stores the throttle speed. As the speed is only set intermittently,
      | the speed is saved to memory and constrantly output. It is only updated when
      | a properly packaged CAN message is delivered based on its ID and the trigger
      | bit.
  In1 : Inport
  Bus Selector2 : BusSelector  OutputSignals=identifier,trigger,data
  Data Store Memory : DataStoreMemory  DataStoreName=throttle_speed  WriteAfterWriteMsg=warning  WriteAfterReadMsg=warning  OutDataTypeStr=double
  Data Store Read : DataStoreRead  Priority=2  DataStoreName=throttle_speed  SampleTime=T_step
  Data Type Conversion : DataTypeConversion  OutDataTypeStr=uint32  RndMeth=Simplest
  If : If  NumInputs=2  IfExpression=u1 == hex2dec('301')  ShowElse=off
  If Action Subsystem : Subsystem  Priority=1  TreatAsAtomicUnit=on
  To Workspace : ToWorkspace  VariableName=t_data  SampleTime=-1  SaveFormat=Structure
  Out1 : Outport
  wires:
  In1/1 -> Bus Selector2/1
  Data Store Read/1 -> Out1/1
  Bus Selector2/1 -> If/1  "<identifier>"
  Bus Selector2/2 -> Data Type Conversion/1  "<trigger>"
  If/1 -> If Action Subsystem/Action
  Bus Selector2/3 -> If Action Subsystem/1(In1), To Workspace/1  "<data>"
  Data Type Conversion/1 -> If/2

== system Boat_sim/Plant/Actuator Dynamics/Subsystem1 ==
  note: This block simulates the stepper motor driver board logic for stepping the motor.
      | The enable line must be low, it's active low, and a pulse train must be received. As
      | the enable line is always low to provide holding torque, the lines specifying a pulse
      | train must are therefore checked to confirm that the rudder should be moving. The
      | exact values of both the up and period signals are unimportant, so they're just
      | compared to zero.
  e : Inport
  u : Inport  Port=2
  p : Inport  Port=3
  Compare To Zero : simulink/Logic and Bit Operations/Compare To Zero  relop=~=  OutDataTypeStr=boolean
  Compare To Zero1 : simulink/Logic and Bit Operations/Compare To Zero  relop=~=  OutDataTypeStr=boolean
  Logical Operator : Logic  Operator=NOT  AllPortsSameDT=off  OutDataTypeStr=boolean
  Logical Operator1 : Logic  Inputs=3  AllPortsSameDT=off  OutDataTypeStr=boolean
  Out1 : Outport
  wires:
  e/1 -> Logical Operator/1
  Logical Operator1/1 -> Out1/1
  p/1 -> Compare To Zero/1
  Compare To Zero/1 -> Logical Operator1/3
  Compare To Zero1/1 -> Logical Operator1/2
  u/1 -> Compare To Zero1/1
  Logical Operator/1 -> Logical Operator1/1

== system Boat_sim/Plant/Forces & Moments/Convert actuator data to heading and speed ==
  Throttle : Inport
  RudderAngle : Inport  Port=2
  Constant4 : Constant  Value=2*pi
  Convert to m/s : Gain  Gain=2.3
  Discrete-Time Integrator : DiscreteIntegrator  SampleTime=.01  ICPrevOutput=DiscIntNeverNeededParam  ICPrevScaledInput=DiscIntNeverNeededParam
  Divide by wheelbase : Gain  Gain=1/wheelbase
  Initial heading : Constant  Value=phi_0
  Math Function : Math  Operator=mod  SaturateOnIntegerOverflow=on
  Negate rudder angle : Gain  Gain=-1
  Product3 : Product  RndMeth=Zero
  Sum2 : Sum  OutDataTypeStr=double
  Trigonometric Function2 : Trigonometry  Operator=tan  OutputSignalType=real
  Speed : Outport
  Heading : Outport  Port=2
  wires:
  Convert to m/s/1 -> Product3/1, Speed/1
  Trigonometric Function2/1 -> Product3/2
  Product3/1 -> Divide by wheelbase/1
  Divide by wheelbase/1 -> Discrete-Time Integrator/1
  Discrete-Time Integrator/1 -> Sum2/1
  Initial heading/1 -> Sum2/2
  Sum2/1 -> Math Function/1
  Negate rudder angle/1 -> Trigonometric Function2/1
  Constant4/1 -> Math Function/2
  Throttle/1 -> Convert to m/s/1
  RudderAngle/1 -> Negate rudder angle/1
  Math Function/1 -> Heading/1

== system Boat_sim/Plant/Forces & Moments/Subsystem ==
  Speed : Inport
  Heading : Inport  Port=2
  Constant : Constant  Value=0
  Discrete-Time Integrator1 : DiscreteIntegrator  SampleTime=-1  UpperSaturationLimit=1  LowerSaturationLimit=-1  ICPrevOutput=DiscIntNeverNeededParam  ICPrevScaledInput=DiscIntNeverNeededParam
  Matrix Concatenate : Concatenate  NumInputs=3  Mode=Vector
  Product1 : Product  RndMeth=Zero
  Product2 : Product  RndMeth=Zero
  Trigonometric Function1 : Trigonometry  OutputSignalType=real
  Trigonometric Function3 : Trigonometry  Operator=cos  OutputSignalType=real
  Position : Outport
  Velocity : Outport  Port=2
  wires:
  Speed/1 -> Product1/1, Product2/1
  Trigonometric Function3/1 -> Product2/2
  Matrix Concatenate/1 -> Discrete-Time Integrator1/1, Velocity/1
  Product2/1 -> Matrix Concatenate/1
  Product1/1 -> Matrix Concatenate/2
  Trigonometric Function1/1 -> Product1/2
  Constant/1 -> Matrix Concatenate/3
  Heading/1 -> Trigonometric Function3/1, Trigonometric Function1/1
  Discrete-Time Integrator1/1 -> Position/1

== system Boat_sim/Plant/Generate sensor data from actuator position/Map from +-.7854 to [347:655] ==
  In1 : Inport
  Bias1 : Bias  Bias=501
  Data Type Conversion : DataTypeConversion  OutDataTypeStr=uint16
  Gain1 : Gain  Gain=-196
  Out1 : Outport
  wires:
  Bias1/1 -> Data Type Conversion/1
  In1/1 -> Gain1/1
  Data Type Conversion/1 -> Out1/1
  Gain1/1 -> Bias1/1

== system Boat_sim/Plant/Generate sensor data from actuator position/Map from -1..1 to -1023..1023 ==
  In1 : Inport
  Data Type Conversion : DataTypeConversion  OutDataTypeStr=int16  RndMeth=Simplest
  Gain : Gain  Gain=1023
  Out1 : Outport
  wires:
  Gain/1 -> Data Type Conversion/1
  In1/1 -> Gain/1
  Data Type Conversion/1 -> Out1/1

== system Boat_sim/Plant/Generate sensor data from actuator position/Map from -1..1 to 620..313 ==
  In1 : Inport
  Bias : Bias  Bias=466.5
  Data Type Conversion : DataTypeConversion  OutDataTypeStr=uint16
  Gain : Gain  Gain=-153.5
  Out1 : Outport
  wires:
  Data Type Conversion/1 -> Out1/1
  In1/1 -> Gain/1
  Bias/1 -> Data Type Conversion/1
  Gain/1 -> Bias/1

== system Boat_sim/Subsystem/Autonomous Controller/Ballast Command ==
  Bus Creator : BusCreator  Inputs=2
  Constant : Constant  Value=0  OutDataTypeStr=boolean
  Constant1 : Constant  Value=0  OutDataTypeStr=boolean
  c_ballast : Outport
  wires:
  Constant1/1 -> Bus Creator/2  "direction"
  Constant/1 -> Bus Creator/1  "enable"
  Bus Creator/1 -> c_ballast/1

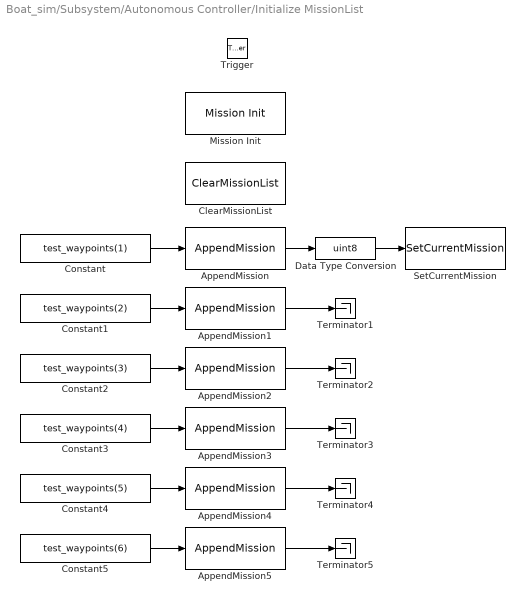
== system Boat_sim/Subsystem/Autonomous Controller/Initialize MissionList ==
  Trigger : TriggerPort  TriggerType=falling  PortDimensions=1
  AppendMission{,1..5} (6 alike) : uSimLib/Mission Manager/AppendMission  sampleTime=-1
  ClearMissionList : uSimLib/Mission Manager/ClearMissionList  Priority=1  sampleTime=-1
      link override Data Store Write1: DataStoreElements=mList.updated
  Constant : Constant  Value=test_waypoints(1)  OutDataTypeStr=Bus: Mission
  Constant1 : Constant  Value=test_waypoints(2)  OutDataTypeStr=Bus: Mission
  Constant2 : Constant  Value=test_waypoints(3)  OutDataTypeStr=Bus: Mission
  Constant3 : Constant  Value=test_waypoints(4)  OutDataTypeStr=Bus: Mission
  Constant4 : Constant  Value=test_waypoints(5)  OutDataTypeStr=Bus: Mission
  Constant5 : Constant  Value=test_waypoints(6)  OutDataTypeStr=Bus: Mission
  Data Type Conversion : DataTypeConversion  OutDataTypeStr=uint8
  Mission Init : uSimLib/Mission Manager/Mission Init  Priority=0  maxMissions=16  sampleTime=-1
      link override Data Store Write: SampleTime=-1
  SetCurrentMission : uSimLib/Mission Manager/SetCurrentMission  sampleTime=-1
  Terminator{1..5} (5 alike) : Terminator
  wires:
  Data Type Conversion/1 -> SetCurrentMission/1
  Constant5/1 -> AppendMission5/1
  AppendMission5/1 -> Terminator5/1
  Constant4/1 -> AppendMission4/1
  AppendMission4/1 -> Terminator4/1
  Constant3/1 -> AppendMission3/1
  AppendMission3/1 -> Terminator3/1
  Constant2/1 -> AppendMission2/1
  AppendMission2/1 -> Terminator2/1
  Constant1/1 -> AppendMission1/1
  AppendMission1/1 -> Terminator1/1
  Constant/1 -> AppendMission/1
  AppendMission/1 -> Data Type Conversion/1
